simulink model "ME425QuadcoptorMotionControl"  (R2024b)
settings: Solver=VariableStepAuto  StartTime=0.0  StopTime=10.0  RelTol=1e-3
undefined symbols (not defined in the file): b, d, g, Ix, Iy, Iz, l, m
settings Model: Creator=Arda Gencer  LastModifiedBy=Arda Gencer

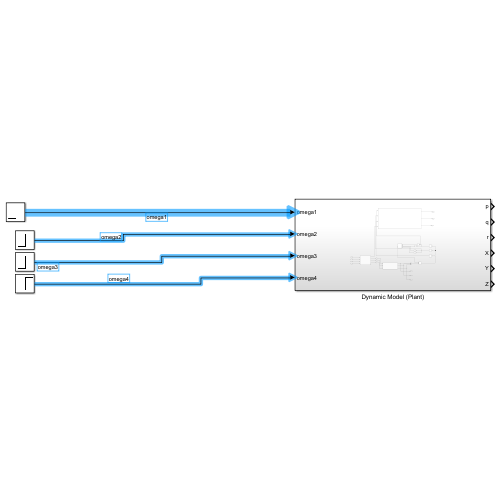
[thumbnail: Simulink's stored preview of the top-level diagram]
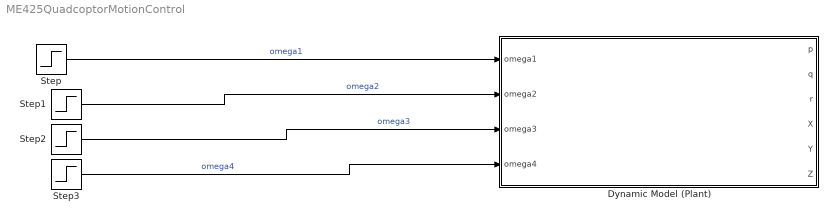
== system ME425QuadcoptorMotionControl ==
  Dynamic Model (Plant) : Subsystem
  Step{,1..3} (4 alike) : Step  SampleTime=0
  wires:
  Step/1 -> Dynamic Model (Plant)/1(omega1)  "omega1"
  Step1/1 -> Dynamic Model (Plant)/2(omega2)  "omega2"
  Step2/1 -> Dynamic Model (Plant)/3(omega3)  "omega3"
  Step3/1 -> Dynamic Model (Plant)/4(omega4)  "omega4"

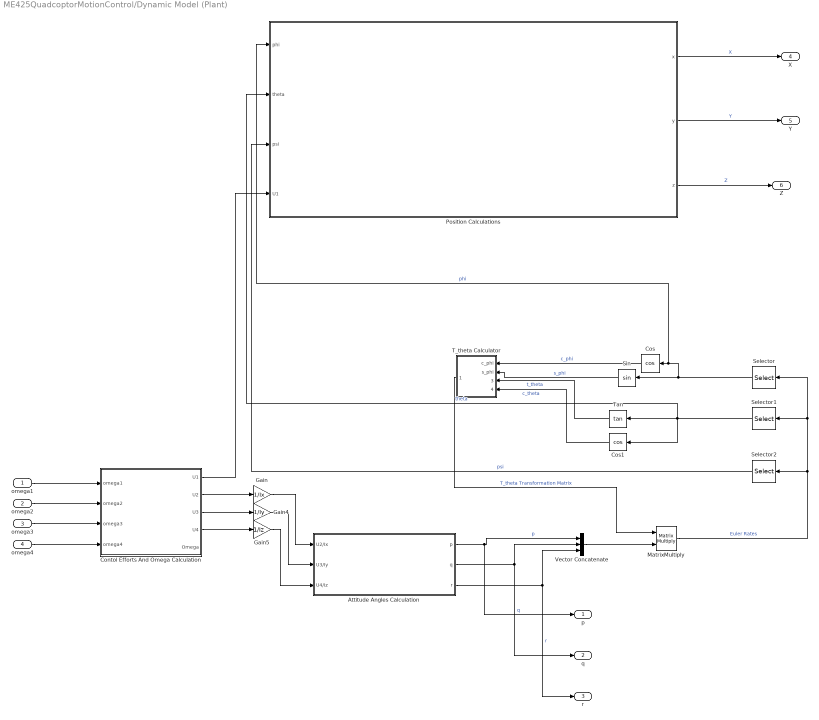
== system ME425QuadcoptorMotionControl/Dynamic Model (Plant) ==
  omega1 : Inport
  omega2 : Inport  Port=2
  omega3 : Inport  Port=3
  omega4 : Inport  Port=4
  Attitude Angles Calculation : Subsystem
  Contol Efforts And Omega Calculation : Subsystem
  Cos : Trigonometry  Operator=cos
  Cos1 : Trigonometry  Operator=cos
  Gain : Gain  Gain=1/Ix
  Gain4 : Gain  Gain=1/Iy
  Gain5 : Gain  Gain=1/Iz
  MatrixMultiply : Product  Multiplication=Matrix(*)
  Position Calculations : Subsystem
  Selector : Selector  InputPortWidth=3  IndexOptions=Index vector (dialog)  Indices=[1]  OutputSizes=1
  Selector1 : Selector  InputPortWidth=3  IndexOptions=Index vector (dialog)  Indices=2  OutputSizes=1
  Selector2 : Selector  InputPortWidth=3  IndexOptions=Index vector (dialog)  Indices=3  OutputSizes=1
  Sin : Trigonometry
  T_theta Calculator : Subsystem
  Tan : Trigonometry  Operator=tan
  Vector Concatenate : Concatenate  NumInputs=3
  p : Outport
  q : Outport  Port=2
  r : Outport  Port=3
  X : Outport  Port=4
  Y : Outport  Port=5
  Z : Outport  Port=6
  wires:
  Vector Concatenate/1 -> MatrixMultiply/2
  Selector1/1 -> Cos1/1, Position Calculations/2(theta), Tan/1  "theta"
  Attitude Angles Calculation/2(q) -> q/1, Vector Concatenate/2  "q"
  Contol Efforts And Omega Calculation/4(U4) -> Gain5/1
  Cos/1 -> T_theta Calculator/1(c_phi)  "c_phi"
  Contol Efforts And Omega Calculation/1(U1) -> Position Calculations/4(U1)
  Selector/1 -> Position Calculations/1(phi), Cos/1, Sin/1  "phi"
  Gain/1 -> Attitude Angles Calculation/1(U2/Ix)
  Gain5/1 -> Attitude Angles Calculation/3(U4/Iz)
  Attitude Angles Calculation/3(r) -> r/1, Vector Concatenate/3  "r"
  Tan/1 -> T_theta Calculator/3(t_theta)  "t_theta"
  Sin/1 -> T_theta Calculator/2(s_phi)  "s_phi"
  Cos1/1 -> T_theta Calculator/4(c_theta)  "c_theta"
  MatrixMultiply/1 -> Selector/1, Selector1/1, Selector2/1  "Euler Rates"
  T_theta Calculator/1(T_theta) -> MatrixMultiply/1  "T_theta Transformation Matrix"
  Contol Efforts And Omega Calculation/2(U2) -> Gain/1
  omega1/1 -> Contol Efforts And Omega Calculation/1(omega1)
  Contol Efforts And Omega Calculation/3(U3) -> Gain4/1
  Selector2/1 -> Position Calculations/3(psi)  "psi"
  Attitude Angles Calculation/1(p) -> p/1, Vector Concatenate/1  "p"
  omega2/1 -> Contol Efforts And Omega Calculation/2(omega2)
  Position Calculations/3(z) -> Z/1  "Z"
  Gain4/1 -> Attitude Angles Calculation/2(U3/Iy)
  omega3/1 -> Contol Efforts And Omega Calculation/3(omega3)
  Position Calculations/1(x) -> X/1  "X"
  Position Calculations/2(y) -> Y/1  "Y"
  omega4/1 -> Contol Efforts And Omega Calculation/4(omega4)

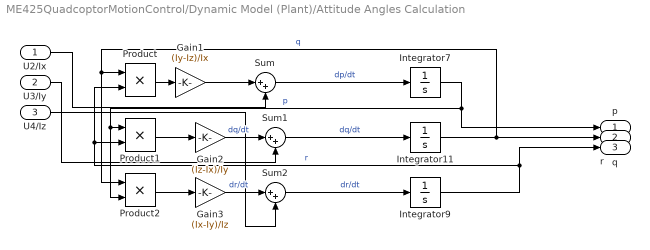
== system ME425QuadcoptorMotionControl/Dynamic Model (Plant)/Attitude Angles Calculation ==
  U2/Ix : Inport
  U3/Iy : Inport  Port=2
  U4/Iz : Inport  Port=3
  Gain1 : Gain  Gain=(Iy-Iz)/Ix
  Gain2 : Gain  Gain=(Iz-Ix)/Iy
  Gain3 : Gain  Gain=(Ix-Iy)/Iz
  Integrator11 : Integrator
  Integrator7 : Integrator
  Integrator9 : Integrator
  Product : Product
  Product1 : Product
  Product2 : Product
  Sum : Sum  Inputs=|++
  Sum1 : Sum  Inputs=|++
  Sum2 : Sum  Inputs=|++
  p : Outport
  q : Outport  Port=2
  r : Outport  Port=3
  wires:
  Integrator11/1 -> q/1, Product2/1, Product/1  "q"
  Integrator7/1 -> p/1, Product2/2, Product1/1  "p"
  Gain1/1 -> Sum/1
  Integrator9/1 -> r/1, Product1/2, Product/2  "r"
  Product2/1 -> Gain3/1
  Sum/1 -> Integrator7/1  "dp/dt"
  Product1/1 -> Gain2/1
  Gain2/1 -> Sum1/1  "dq/dt"
  Gain3/1 -> Sum2/1  "dr/dt"
  Sum1/1 -> Integrator11/1  "dq/dt"
  Sum2/1 -> Integrator9/1  "dr/dt"
  U3/Iy/1 -> Sum1/2
  Product/1 -> Gain1/1
  U2/Ix/1 -> Sum/2
  U4/Iz/1 -> Sum2/2

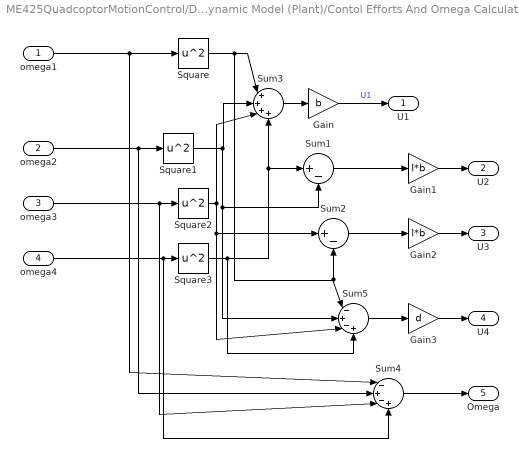
== system ME425QuadcoptorMotionControl/Dynamic Model (Plant)/Contol Efforts And Omega Calculation ==
  omega1 : Inport
  omega2 : Inport  Port=2
  omega3 : Inport  Port=3
  omega4 : Inport  Port=4
  Gain : Gain  Gain=b
  Gain1 : Gain  Gain=l*b
  Gain2 : Gain  Gain=l*b
  Gain3 : Gain  Gain=d
  Square{,1..3} (4 alike) : Math  Operator=square
  Sum1 : Sum  Inputs=|+-
  Sum2 : Sum  Inputs=|+-
  Sum3 : Sum  Inputs=|++++
  Sum4 : Sum  Inputs=|-+-+
  Sum5 : Sum  Inputs=|-+-+
  U1 : Outport
  U2 : Outport  Port=2
  U3 : Outport  Port=3
  U4 : Outport  Port=4
  Omega : Outport  Port=5
  wires:
  omega3/1 -> Sum4/3, Square2/1
  Sum3/1 -> Gain/1
  Square/1 -> Sum5/1, Sum2/2, Sum3/1
  Square1/1 -> Sum5/2, Sum1/2, Sum3/2
  Square2/1 -> Sum5/3, Sum2/1, Sum3/3
  omega4/1 -> Sum4/4, Square3/1
  Square3/1 -> Sum5/4, Sum1/1, Sum3/4
  omega2/1 -> Sum4/2, Square1/1
  omega1/1 -> Sum4/1, Square/1
  Gain/1 -> U1/1  "U1"
  Sum1/1 -> Gain1/1
  Gain1/1 -> U2/1
  Gain2/1 -> U3/1
  Sum2/1 -> Gain2/1
  Gain3/1 -> U4/1
  Sum4/1 -> Omega/1
  Sum5/1 -> Gain3/1

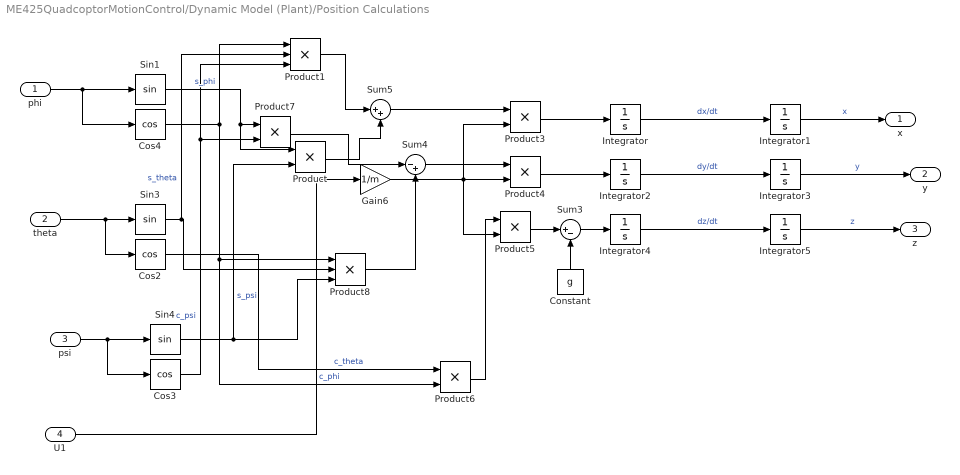
== system ME425QuadcoptorMotionControl/Dynamic Model (Plant)/Position Calculations ==
  phi : Inport
  theta : Inport  Port=2
  psi : Inport  Port=3
  U1 : Inport  Port=4
  Constant : Constant  Value=g
  Cos2 : Trigonometry  Operator=cos
  Cos3 : Trigonometry  Operator=cos
  Cos4 : Trigonometry  Operator=cos
  Gain6 : Gain  Gain=1/m
  Integrator{,1..5} (6 alike) : Integrator
  Product{,3..7} (6 alike) : Product
  Product1 : Product  Inputs=3
  Product8 : Product  Inputs=3
  Sin1 : Trigonometry
  Sin3 : Trigonometry
  Sin4 : Trigonometry
  Sum3 : Sum  Inputs=|+-
  Sum4 : Sum  Inputs=|-+
  Sum5 : Sum  Inputs=|++
  x : Outport
  y : Outport  Port=2
  z : Outport  Port=3
  wires:
  Integrator4/1 -> Integrator5/1  "dz/dt"
  Sin3/1 -> Product1/2, Product8/2  "s_theta"
  psi/1 -> Cos3/1, Sin4/1
  U1/1 -> Gain6/1
  Sum4/1 -> Product4/1
  Integrator2/1 -> Integrator3/1  "dy/dt"
  Cos4/1 -> Product8/1, Product6/2, Product1/1  "c_phi"
  Integrator1/1 -> x/1  "x"
  theta/1 -> Cos2/1, Sin3/1
  Gain6/1 -> Product3/2, Product5/2, Product4/2
  Sum3/1 -> Integrator4/1
  Sin4/1 -> Product/2, Product8/3  "s_psi"
  Product1/1 -> Sum5/1
  Integrator/1 -> Integrator1/1  "dx/dt"
  Sum5/1 -> Product3/1
  Cos3/1 -> Product1/3, Product7/2  "c_psi"
  Product3/1 -> Integrator/1
  Product4/1 -> Integrator2/1
  Cos2/1 -> Product6/1  "c_theta"
  phi/1 -> Cos4/1, Sin1/1
  Product7/1 -> Sum4/1
  Product6/1 -> Product5/1
  Product/1 -> Sum5/2
  Constant/1 -> Sum3/2
  Product5/1 -> Sum3/1
  Sin1/1 -> Product/1, Product7/1  "s_phi"
  Product8/1 -> Sum4/2
  Integrator3/1 -> y/1  "y"
  Integrator5/1 -> z/1  "z"

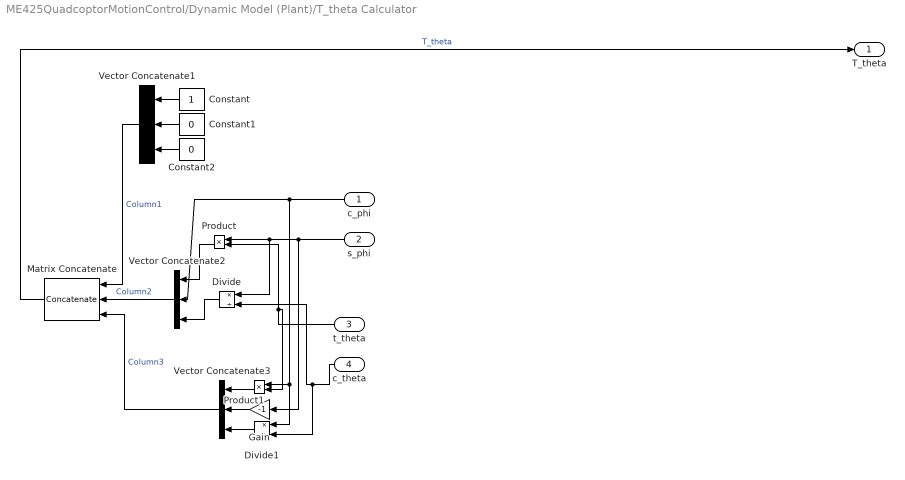
== system ME425QuadcoptorMotionControl/Dynamic Model (Plant)/T_theta Calculator ==
  c_phi : Inport
  s_phi : Inport  Port=2
  t_theta : Inport  Port=3
  c_theta : Inport  Port=4
  Constant : Constant
  Constant1 : Constant  Value=0
  Constant2 : Constant  Value=0
  Divide : Product  Inputs=*/
  Divide1 : Product  Inputs=*/
  Gain : Gain  Gain=-1
  Matrix Concatenate : Concatenate  NumInputs=3  Mode=Multidimensional array  ConcatenateDimension=2
  Product : Product
  Product1 : Product
  Vector Concatenate1 : Concatenate  NumInputs=3
  Vector Concatenate2 : Concatenate  NumInputs=3
  Vector Concatenate3 : Concatenate  NumInputs=3
  T_theta : Outport
  wires:
  c_theta/1 -> Divide/2, Divide1/2
  c_phi/1 -> Vector Concatenate2/2, Divide1/1, Product1/1
  Constant/1 -> Vector Concatenate1/1
  Vector Concatenate2/1 -> Matrix Concatenate/2  "Column2"
  Product/1 -> Vector Concatenate2/1
  s_phi/1 -> Product/1, Divide/1, Gain/1
  Product1/1 -> Vector Concatenate3/1
  Vector Concatenate3/1 -> Matrix Concatenate/3  "Column3"
  Matrix Concatenate/1 -> T_theta/1  "T_theta"
  Constant2/1 -> Vector Concatenate1/3
  Constant1/1 -> Vector Concatenate1/2
  Vector Concatenate1/1 -> Matrix Concatenate/1  "Column1"
  t_theta/1 -> Product1/2, Product/2
  Gain/1 -> Vector Concatenate3/2
  Divide1/1 -> Vector Concatenate3/3
  Divide/1 -> Vector Concatenate2/3
